simulink model "R7014E_QuadTankSim_With_Kalman"  (R2018b)
settings: Solver=VariableStepAuto  StartTime=0.0  StopTime=1000  RelTol=1e-3
values from neighbouring files (symbols this model uses):
  A = 33    [Lab1.m]    (also in LabB_FInal_version2.mat; Untitled.m)
  C = [C1;C2]    [Lab1.m]    (also in LabB_FInal_version2.mat = [1  0; 0  1]; Untitled.m)
undefined symbols (not defined in the file or in its folder): B, Continuous, D, sigbuilder_block, Time
libraries: simulink x1, ctrlSharedLib x1, cstblocks x1
settings Model: NumberOfSteps=100  Creator=OscarBackman  LastModifiedBy=OscarBackman

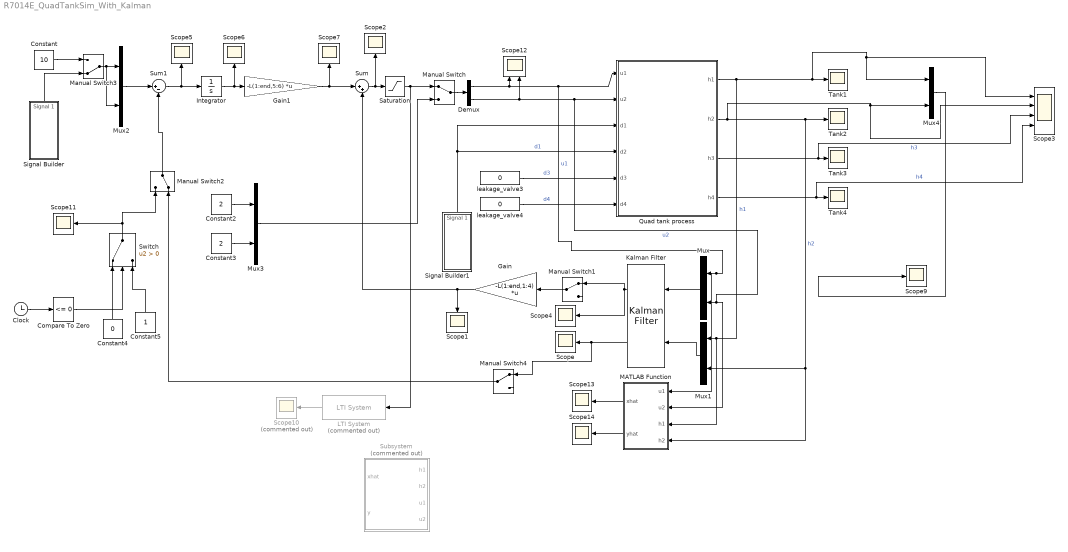
== system R7014E_QuadTankSim_With_Kalman ==
  Clock : Clock
      settings: Decimation=10000
  Compare To Zero : simulink/Logic and Bit Operations/Compare To Zero  relop=<=  OutDataTypeStr=boolean
  Constant : Constant  Value=10
  Constant2 : Constant  Value=2
  Constant3 : Constant  Value=2
  Constant4 : Constant  Value=0
  Constant5 : Constant
  Demux : Demux  Outputs=2
  Gain : Gain  Gain=-L(1:end,1:4)  Multiplication=Matrix(K*u)
  Gain1 : Gain  Gain=-L(1:end,5:6)  Multiplication=Matrix(K*u)
  Integrator : Integrator
  Kalman Filter : ctrlSharedLib/Kalman Filter  TimeDomain=Continuous-Time  UseCurrentEstimator=on  ModelSource=Individual A, B, C, D matrices  ModelSourceVariable=ss(0.95,1,1,0,1)  A=A  B=B  C=C  D=D  NumberOfStates=4  NumberOfInputs=2  NumberOfOutputs=4  InitialEstimateSource=Dialog  X0=[0 0 0 0]  P0=10  UseK=off  UseGH=off  NumberOfProcessNoiseInputs=1  G=1  TimeInvariantG=on  H=0  TimeInvariantH=on  Q=1  TimeInvariantQ=on  R=1  TimeInvariantR=on  N=0  TimeInvariantN=on  AddInputPort=on  AddEnablePort=off  OutputEstimatedY=on  OutputP=off  Ts=-1
      settings: SourceProductBaseCode=CT
  LTI System : cstblocks/LTI System  Commented=on  sys=G  IC=[]
  MATLAB Function : MATLAB Function  TreatAsAtomicUnit=on
  Manual Switch : ManualSwitch
  Manual Switch1 : ManualSwitch
  Manual Switch2 : ManualSwitch  CurrentSetting=0
  Manual Switch3 : ManualSwitch  CurrentSetting=0
  Manual Switch4 : ManualSwitch
  Mux{,1..4} (5 alike) : Mux  Inputs=2
  Quad tank process : Subsystem  mask{hmax=20, A1=28, ao1=0.071, h10=0, A2=32, ao2=0.057, h20=0, A3=28, ao3=0.071, h30=0, A4=32, ao4=0.057, h40=0, k1=3.33, k2=3.35, gamma1=0.7, gamma2=0.6}
      mask prompts: hmax "Tank height (cm)"; A1 "Tank area (cm^2)"; ao1 "Opening area (cm^2)"; h10 "Initial level (cm)"; A2 "Tank area (cm^2)"; ao2 "Opening area (cm^2)"; h20 "Initial level (cm)"; A3 "Tank area (cm^2)"; ao3 "Opening area (cm^2)"; h30 "Initial level (cm)"; A4 "Tank area (cm^2)"; ao4 "Opening area (cm^2)"; h40 "Initial level (cm)"; k1 "Pump1 gain (cm^3/V/s)"; k2 "Pump2 gain (cm^3/V/s)"; gamma1 "Split valve gamma 1"; gamma2 "Split valve gamma 2"
      mask help: Double tank process parameters
      mask DialogControl Container3 Prompt: General parameters
      mask DialogControl ParameterGroupVar Prompt: Tank 1
      mask DialogControl ParameterGroupVar_copy_copy_copy Prompt: Tank 2
      mask DialogControl ParameterGroupVar_copy_copy Prompt: Tank 3
      mask DialogControl ParameterGroupVar_copy Prompt: Tank 4
      mask DialogControl Container4 Prompt: Pump parameters
  Saturation : Saturate  UpperLimit=10  LowerLimit=0
  Scope{,1..2,4..7,9,11,13..14} (11 alike) : Scope
  Scope10 : Scope  Commented=on
  Scope12 : Scope  NumInputPorts=2
  Scope3 : Scope  NumInputPorts=4
  Signal Builder : Subsystem  Tag=STV Subsys  LoadFcn=sigbuilder_block('load');  StartFcn=sigbuilder_block('start');  StopFcn=sigbuilder_block('stop');  ClipboardFcn=sigbuilder_block('clipboard');  mask(Sigbuilder block){tuvar=[0:10]}
      mask help: Simulink:masks:SigbuilderBlock_MD
      mask init:
      | if ~strcmp(get_param(bdroot(gcbh),'SimulationStatus'),'stopped') tuvar = sigbuilder_block('maskInit'); end
      settings: CopyFcn=sigbuilder_block('copy');  DeleteFcn=sigbuilder_block('delete');  ModelCloseFcn=sigbuilder_block('modelClose');  PreSaveFcn=sigbuilder_block('preSave');  PauseFcn=sigbuilder_block('pause');  ContinueFcn=sigbuilder_block('continue');  NameChangeFcn=sigbuilder_block('namechange');  OpenFcn=sigbuilder_block('open',[437.6 180 550.4 400.2 ]);  CloseFcn=sigbuilder_block('close');
      mask Display: plot(0, 0, 100, 100,[2, 2, 32, 32, 2], [68, 8, 8, 68, 68],[32, 2], [38, 38], [32, 19, 2],[53, 60, 44], [32, 17, 17, 2],[16, 16, 31, 31]);txt = getActiveGroup(gcbh);text(2, 100, txt,'verticalAlignment', 'top');
  Signal Builder1 : Subsystem  Tag=STV Subsys  LoadFcn=sigbuilder_block('load');  StartFcn=sigbuilder_block('start');  StopFcn=sigbuilder_block('stop');  ClipboardFcn=sigbuilder_block('clipboard');  mask(Sigbuilder block){tuvar=[0:10]}
      mask help: Simulink:masks:SigbuilderBlock_MD
      mask init:
      | if ~strcmp(get_param(bdroot(gcbh),'SimulationStatus'),'stopped') tuvar = sigbuilder_block('maskInit'); end
      settings: CopyFcn=sigbuilder_block('copy');  DeleteFcn=sigbuilder_block('delete');  ModelCloseFcn=sigbuilder_block('modelClose');  PreSaveFcn=sigbuilder_block('preSave');  PauseFcn=sigbuilder_block('pause');  ContinueFcn=sigbuilder_block('continue');  NameChangeFcn=sigbuilder_block('namechange');  OpenFcn=sigbuilder_block('open',[437.6 180 550.4 400.2 ]);  CloseFcn=sigbuilder_block('close');
      mask Display: plot(0, 0, 100, 100,[2, 2, 32, 32, 2], [68, 8, 8, 68, 68],[32, 2], [38, 38], [32, 19, 2],[53, 60, 44], [32, 17, 17, 2],[16, 16, 31, 31]);txt = getActiveGroup(gcbh);text(2, 100, txt,'verticalAlignment', 'top');
  Subsystem : Subsystem  Commented=on
  Sum : Sum  Inputs=|++
  Sum1 : Sum  Inputs=|+-
  Switch : Switch  Criteria=u2 > Threshold
  Tank{1..4} (4 alike) : Scope
  leakage_valve3 : Constant  Value=0
  leakage_valve4 : Constant  Value=0
  wires:
  leakage_valve4/1 -> Quad tank process/6(d4)  "d4"
  Quad tank process/2(h2) -> MATLAB Function/4(h2), Mux1/2, Tank2/1, Scope3/2, Mux4/2  "h2"
  Quad tank process/1(h1) -> MATLAB Function/3(h1), Mux1/1, Mux4/1, Scope3/1, Tank1/1  "h1"
  leakage_valve3/1 -> Quad tank process/5(d3)  "d3"
  Signal Builder1/1(Signal 1) -> Quad tank process/3(d1), Quad tank process/4(d2)  "d1"
  Quad tank process/4(h4) -> Scope3/4, Tank4/1  "h4"
  Quad tank process/3(h3) -> Scope3/3, Tank3/1  "h3"
  Mux/1 -> Kalman Filter/1
  Mux1/1 -> Kalman Filter/2
  Kalman Filter/1 -> Scope4/1, Manual Switch1/1
  Demux/1 -> Scope12/1, Quad tank process/1(u1), MATLAB Function/1(u1), Mux/1  "u1"
  Demux/2 -> Scope12/2, Quad tank process/2(u2), MATLAB Function/2(u2), Mux/2  "u2"
  Constant3/1 -> Mux3/2
  Constant2/1 -> Mux3/1
  Manual Switch/1 -> Demux/1
  Sum/1 -> Scope2/1, Saturation/1
  Gain/1 -> Sum/2, Scope1/1
  Manual Switch1/1 -> Gain/1
  Mux2/1 -> Sum1/1
  Sum1/1 -> Integrator/1, Scope5/1
  Gain1/1 -> Scope7/1, Sum/1
  Integrator/1 -> Scope6/1, Gain1/1
  Mux3/1 -> Manual Switch/2
  Saturation/1 -> Manual Switch/1, LTI System/1
  Kalman Filter/2 -> Manual Switch4/1, Scope/1
  Manual Switch2/1 -> Sum1/2
  Switch/1 -> Manual Switch2/1, Scope11/1
  Clock/1 -> Compare To Zero/1
  Constant4/1 -> Switch/1
  LTI System/1 -> Scope10/1
  Manual Switch3/1 -> Mux2/2, Mux2/1
  Signal Builder/1(Signal 1) -> Manual Switch3/2
  Constant/1 -> Manual Switch3/1
  Compare To Zero/1 -> Switch/2
  Mux4/1 -> Scope9/1
  Constant5/1 -> Switch/3
  MATLAB Function/1(xhat) -> Scope13/1
  MATLAB Function/2(yhat) -> Scope14/1
  Manual Switch4/1 -> Manual Switch2/2

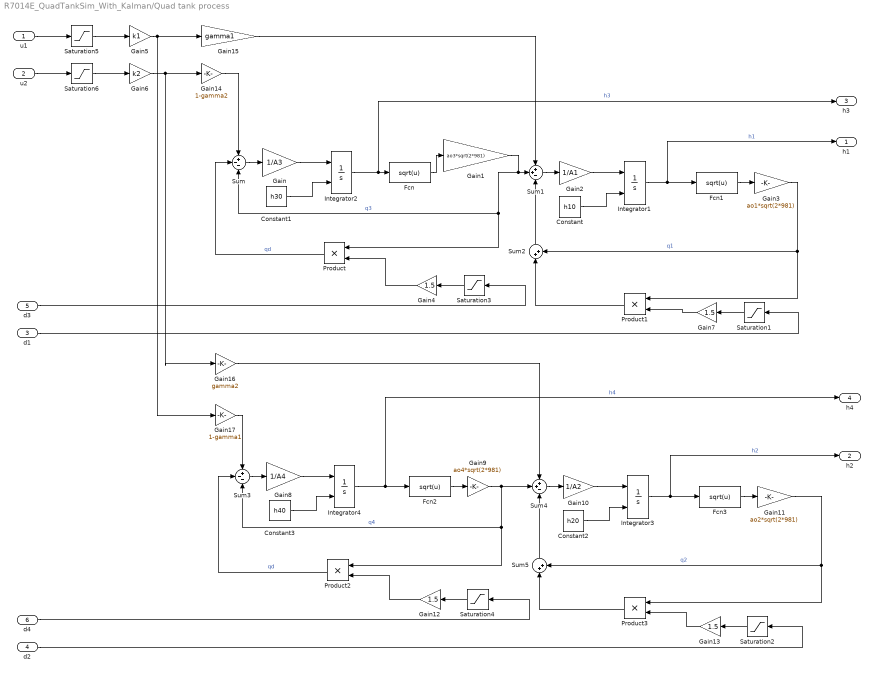
== system R7014E_QuadTankSim_With_Kalman/Quad tank process ==
  u1 : Inport
  u2 : Inport  Port=2
  d1 : Inport  Port=3
  d2 : Inport  Port=4
  d3 : Inport  Port=5
  d4 : Inport  Port=6
  Constant : Constant  Value=h10
  Constant1 : Constant  Value=h30
  Constant2 : Constant  Value=h20
  Constant3 : Constant  Value=h40
  Fcn{,1..3} (4 alike) : Fcn  Expr=sqrt(u)
  Gain : Gain  Gain=1/A3
  Gain1 : Gain  Gain=ao3*sqrt(2*981)
  Gain10 : Gain  Gain=1/A2
  Gain11 : Gain  Gain=ao2*sqrt(2*981)
  Gain{4,7,12..13} (4 alike) : Gain  Gain=1.5
  Gain14 : Gain  Gain=1-gamma2
  Gain15 : Gain  Gain=gamma1
  Gain16 : Gain  Gain=gamma2
  Gain17 : Gain  Gain=1-gamma1
  Gain2 : Gain  Gain=1/A1
  Gain3 : Gain  Gain=ao1*sqrt(2*981)
  Gain5 : Gain  Gain=k1
  Gain6 : Gain  Gain=k2
  Gain8 : Gain  Gain=1/A4
  Gain9 : Gain  Gain=ao4*sqrt(2*981)
  Integrator{1..4} (4 alike) : Integrator  InitialConditionSource=external  LimitOutput=on  UpperSaturationLimit=hmax  LowerSaturationLimit=0
  Product{,1..3} (4 alike) : Product  RndMeth=Zero
  Saturation{1..4} (4 alike) : Saturate  UpperLimit=1  LowerLimit=0
  Saturation5 : Saturate  UpperLimit=10  LowerLimit=0
  Saturation6 : Saturate  UpperLimit=10  LowerLimit=0
  Sum : Sum  Inputs=+--
  Sum1 : Sum  Inputs=++-
  Sum2 : Sum  Inputs=|++
  Sum3 : Sum  Inputs=+--
  Sum4 : Sum  Inputs=++-
  Sum5 : Sum  Inputs=|++
  h1 : Outport
  h2 : Outport  Port=2
  h3 : Outport  Port=3
  h4 : Outport  Port=4
  wires:
  Sum/1 -> Gain/1
  Gain/1 -> Integrator2/1
  Fcn/1 -> Gain1/1
  Gain1/1 -> Product/1, Sum/3, Sum1/2  "q3"
  Sum1/1 -> Gain2/1
  Gain2/1 -> Integrator1/1
  Fcn1/1 -> Gain3/1
  Integrator2/1 -> h3/1, Fcn/1  "h3"
  Product/1 -> Sum/2  "qd"
  d3/1 -> Saturation3/1
  Integrator1/1 -> h1/1, Fcn1/1  "h1"
  Saturation3/1 -> Gain4/1
  Gain4/1 -> Product/2
  u1/1 -> Saturation5/1
  Constant/1 -> Integrator1/2
  Constant1/1 -> Integrator2/2
  u2/1 -> Saturation6/1
  Gain5/1 -> Gain17/1, Gain15/1
  Sum2/1 -> Sum1/3
  Gain3/1 -> Product1/1, Sum2/2  "q1"
  Gain7/1 -> Product1/2
  Saturation1/1 -> Gain7/1
  d1/1 -> Saturation1/1
  Product1/1 -> Sum2/1
  Product3/1 -> Sum5/1
  d2/1 -> Saturation2/1
  Saturation2/1 -> Gain13/1
  Gain13/1 -> Product3/2
  Gain11/1 -> Sum5/2, Product3/1  "q2"
  Sum5/1 -> Sum4/3
  Constant3/1 -> Integrator4/2
  Constant2/1 -> Integrator3/2
  Gain12/1 -> Product2/2
  Saturation4/1 -> Gain12/1
  Integrator3/1 -> Fcn3/1, h2/1  "h2"
  d4/1 -> Saturation4/1
  Product2/1 -> Sum3/2  "qd"
  Integrator4/1 -> h4/1, Fcn2/1  "h4"
  Fcn3/1 -> Gain11/1
  Gain10/1 -> Integrator3/1
  Sum4/1 -> Gain10/1
  Gain9/1 -> Sum4/2, Sum3/3, Product2/1  "q4"
  Fcn2/1 -> Gain9/1
  Gain8/1 -> Integrator4/1
  Sum3/1 -> Gain8/1
  Gain14/1 -> Sum/1
  Gain15/1 -> Sum1/1
  Gain6/1 -> Gain16/1, Gain14/1
  Gain16/1 -> Sum4/1
  Gain17/1 -> Sum3/1
  Saturation5/1 -> Gain5/1
  Saturation6/1 -> Gain6/1

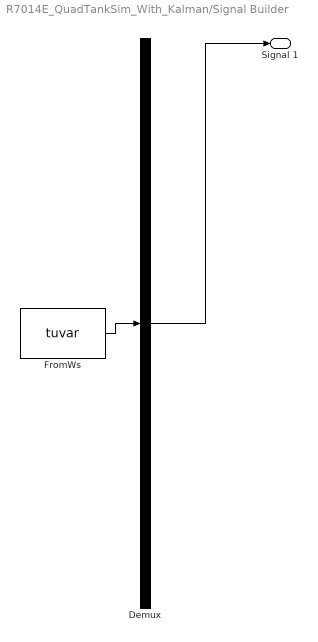
== system R7014E_QuadTankSim_With_Kalman/Signal Builder ==
  Demux : Demux  Tag=STV Demux  Outputs=1
  FromWs : FromWorkspace  Tag=STV FromWs  VariableName=tuvar  SampleTime=0
      SigBuilderData=|
      | common.afterFinalStr = 'Extrapolate'
      | common.sampleTime = 0
      | dataSet.timeRange = [0 1000]
      | dataSet.name = 'Group 1'
      | sbobj.Groups.Name = 'Group 1'
      | sbobj.Groups.Signals.Name = 'Signal 1'
      | sbobj.Groups.Signals.XData = [0 500 500 1000]
      | sbobj.Groups.Signals.YData = [10 10 12 12]
      | sbobj.Groups.TimeRange = [0 1000]
  Signal 1 : Outport  Tag=STV Outport
  wires:
  Demux/1 -> Signal 1/1
  FromWs/1 -> Demux/1

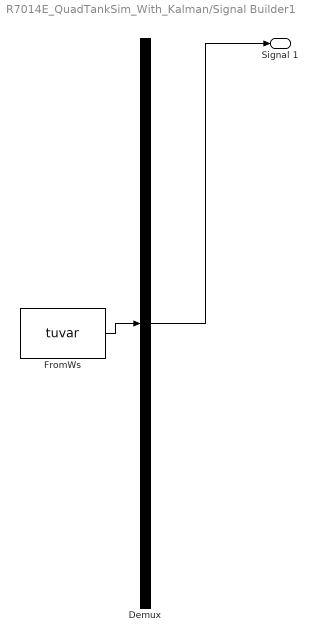
== system R7014E_QuadTankSim_With_Kalman/Signal Builder1 ==
  Demux : Demux  Tag=STV Demux  Outputs=1
  FromWs : FromWorkspace  Tag=STV FromWs  VariableName=tuvar  SampleTime=0
      SigBuilderData=|
      | common.afterFinalStr = 'Extrapolate'
      | common.sampleTime = 0
      | dataSet.timeRange = [0 1000]
      | dataSet.name = 'Group 1'
      | sbobj.Groups.Name = 'Group 1'
      | sbobj.Groups.Signals.Name = 'Signal 1'
      | sbobj.Groups.Signals.XData = [0 700 700 1000]
      | sbobj.Groups.Signals.YData = [0 0 0.25 0.25]
      | sbobj.Groups.TimeRange = [0 1000]
  Signal 1 : Outport  Tag=STV Outport
  wires:
  Demux/1 -> Signal 1/1
  FromWs/1 -> Demux/1

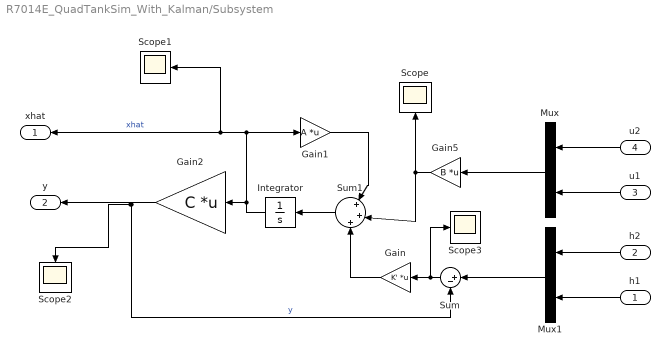
== system R7014E_QuadTankSim_With_Kalman/Subsystem ==
  h1 : Inport
  h2 : Inport  Port=2
  u1 : Inport  Port=3
  u2 : Inport  Port=4
  Gain : Gain  Gain=K'  Multiplication=Matrix(K*u)
  Gain1 : Gain  Gain=A  Multiplication=Matrix(K*u)
  Gain2 : Gain  Gain=C  Multiplication=Matrix(K*u)
  Gain5 : Gain  Gain=B  Multiplication=Matrix(K*u)
  Integrator : Integrator
  Mux : Mux  Inputs=2
  Mux1 : Mux  Inputs=2
  Scope{,1..3} (4 alike) : Scope
  Sum : Sum  Inputs=|+-
  Sum1 : Sum  Inputs=|+|+|+
  xhat : Outport
  "y " : Outport  Port=2
  wires:
  h2/1 -> Mux1/1
  h1/1 -> Mux1/2
  u1/1 -> Mux/2
  u2/1 -> Mux/1
  Gain5/1 -> Sum1/2, Scope/1
  Mux/1 -> Gain5/1
  Mux1/1 -> Sum/1
  Sum/1 -> Scope3/1, Gain/1
  Gain/1 -> Sum1/3
  Sum1/1 -> Integrator/1
  Integrator/1 -> Gain2/1, xhat/1, Scope1/1, Gain1/1  "xhat"
  Gain1/1 -> Sum1/1
  Gain2/1 -> Sum/2, "y "/1, Scope2/1  "y"

== matlab function R7014E_QuadTankSim_With_Kalman/MATLAB Function ==
  settings: updateMethod=DISCRETE
  data: xhat output; u1 input; yhat output; u2 input; h1 input; h2 input
function [xhat,yhat] = fcn(u1,u2,h1,h2)

A = [-0.0209    0.0172    0.0099   -0.0007;
   -0.0016   -0.0635   -0.0300   -0.0015;
    0.0012    0.0187   -0.0161    0.0012;
    0.0271   -0.0034   -0.0182   -0.0348]
B = [
    0.1319    0.0407;
   -0.0934    0.0611;
    0.0735    0.0503;
   -0.1178    0.2137]
C = [0.0754   -0.0394    0.2728   -0.0673
    0.1121   -0.0000    0.0000    0.1256]

K = [
    0.2224   -0.0153    0.9320   -0.1985;
    0.7624    0.0722   -0.0568    0.5817]'


 persistent x 
 
 
 if isempty(x)          %undefined
      x= [0;0;0;0];
      
 end


x = A*x +B*[u1 u2]'      %+K*([h1 h2]'-yhat)
yhat = C*x


xhat = 

end
